simulink model "optimpid_OL_simuink"  (Simulink 10.1)
settings: Solver=ode45  StartTime=0.0  StopTime=10.0  RelTol=1e-3  EnableMultiTasking=on
undefined symbols (not defined in the file or in its folder): den_G_R_V, den_st, num_G_R_V, num_st
settings Model: Creator=Professor Dingyu Xue  LastModifiedBy=msi
settings DataIOCC: LimitDataPoints=on  SignalLoggingSaveFormat=ModelDataLogs
settings OptimizationCC: DefaultParameterBehavior=Inlined  ExpressionDepthLimit=2147483647
settings DebuggingCC: SolverPrmCheckMsg=warning  FcnCallInpInsideContextMsg=warning  StateNameClashWarn=warning

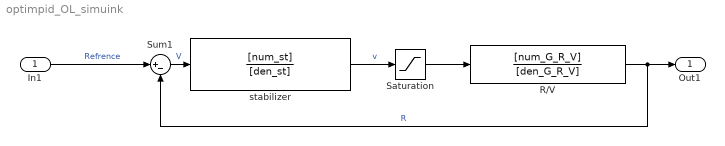
== system optimpid_OL_simuink ==
  In1 : Inport
  R/V : TransferFcn  Numerator=[num_G_R_V]  Denominator=[den_G_R_V]
  Saturation : Saturate  UpperLimit=10  LowerLimit=-10
  Sum1 : Sum  Inputs=|+-
  stabilizer : TransferFcn  Numerator=[num_st]  Denominator=[den_st]
  Out1 : Outport
  wires:
  Sum1/1 -> stabilizer/1  "V"
  stabilizer/1 -> Saturation/1  "v"
  R/V/1 -> Out1/1, Sum1/2  "R"
  In1/1 -> Sum1/1  "Refrence"
  Saturation/1 -> R/V/1
